simulink model "mode_select_lib_test"  (R2018b)
settings: Solver=VariableStepAuto  StartTime=0.0  StopTime=300000  RelTol=1e-3
undefined symbols (not defined in the file): simParams
libraries: CDH_command_lib x1, mode_select_lib x1
settings Model: Creator=taylorreynolds  LastModifiedBy=sophiakim

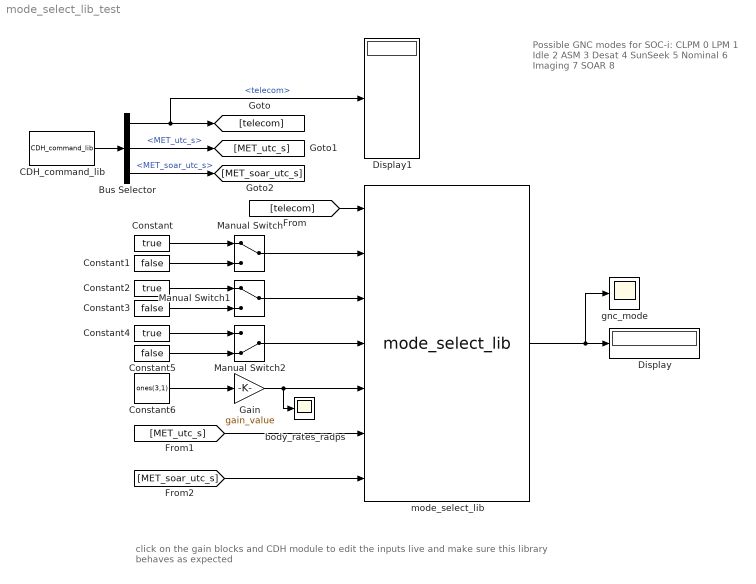
== system mode_select_lib_test ==
  note: click on the gain blocks and CDH module to edit the inputs live and make sure
      | this library behaves as expected
  note: Possible GNC modes for SOC-i:
      | CLPM 0
      | LPM 1
      | Idle 2
      | ASM 3
      | Desat 4
      | SunSeek 5
      | Nominal 6
      | Imaging 7
      | SOAR 8
  Bus Selector : BusSelector  OutputSignals=telecom,MET_utc_s,MET_soar_utc_s
  CDH_command_lib : CDH_command_lib/CDH_command_lib  target_lat_deg=47  target_lon_deg=-122  target_alt_m=44  override_autonomy=0  enable_pointing=on  force_clpm=off  force_lpm=off  enable_img=on  enable_soar=off  triad_override=off  MET_soar_utc_s=simParams.time.epoch_utc_s+2000  quat_soar_cmd=[1;0;0;0]
  Constant : Constant  Value=true
  Constant1 : Constant  Value=false
  Constant2 : Constant  Value=true
  Constant3 : Constant  Value=false
  Constant4 : Constant  Value=true
  Constant5 : Constant  Value=false
  Constant6 : Constant  Value=ones(3,1)
  Display : Display
  Display1 : Display
  Gain : Gain  Gain=gain_value  mask{gain_value=0}
      mask prompts: gain_value "Gain"
  Manual Switch : ManualSwitch
  Manual Switch1 : ManualSwitch
  Manual Switch2 : ManualSwitch  CurrentSetting=0
  body_rates_radps : Scope
  gnc_mode : Scope
  mode_select_lib : mode_select_lib/mode_select_lib  SystemSampleTime=-1
  wires:
  mode_select_lib/1 -> gnc_mode/1, Display/1
  CDH_command_lib/1 -> Bus Selector/1
  Manual Switch/1 -> mode_select_lib/2
  Constant/1 -> Manual Switch/1
  Constant1/1 -> Manual Switch/2
  Constant3/1 -> Manual Switch1/2
  Constant2/1 -> Manual Switch1/1
  Manual Switch1/1 -> mode_select_lib/3
  Manual Switch2/1 -> mode_select_lib/4
  Constant4/1 -> Manual Switch2/1
  Constant5/1 -> Manual Switch2/2
  Constant6/1 -> Gain/1
  Bus Selector/2 -> [MET_utc_s]  "<MET_utc_s>"
  Bus Selector/1 -> Display1/1, [telecom]  "<telecom>"
  [telecom] -> mode_select_lib/1
  [MET_utc_s] -> mode_select_lib/6
  Gain/1 -> body_rates_radps/1, mode_select_lib/5
  Bus Selector/3 -> [MET_soar_utc_s]  "<MET_soar_utc_s>"
  [MET_soar_utc_s] -> mode_select_lib/7
